simulink model "carga_on_off"  (R2024b)
settings: Solver=VariableStepAuto  StartTime=0.0  StopTime=10.0  RelTol=1e-3
undefined symbols (not defined in the file): bc_x, bc_y, H_c, Kc_y, M_s, M_x
settings Model: Creator=ribei  LastModifiedBy=ribei

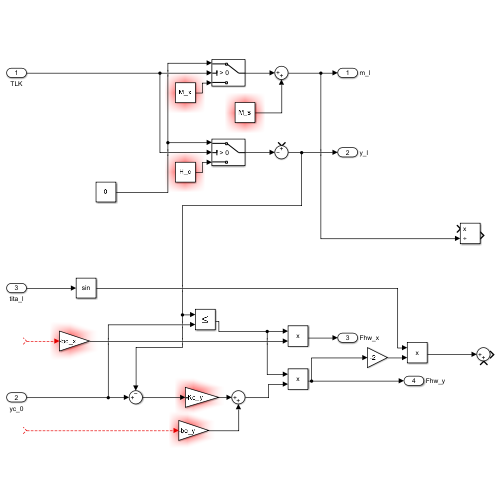
[thumbnail: Simulink's stored preview of the top-level diagram]
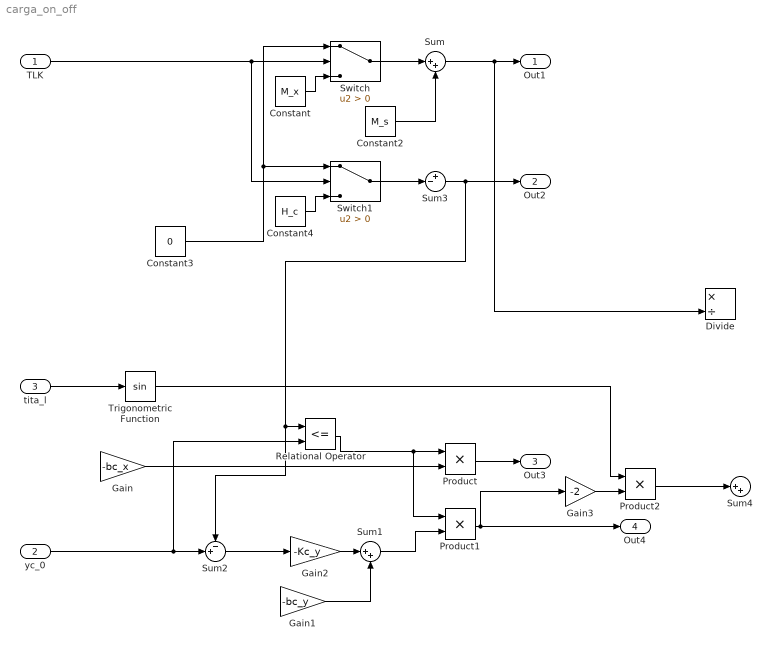
== system carga_on_off ==
  TLK : Inport
  yc_0 : Inport  Port=2
  tita_l : Inport  Port=3
  Constant : Constant  Value=M_x
  Constant2 : Constant  Value=M_s
  Constant3 : Constant  Value=0
  Constant4 : Constant  Value=H_c
  Divide : Product  Inputs=*/
  Gain : Gain  Gain=-bc_x
  Gain1 : Gain  Gain=-bc_y
  Gain2 : Gain  Gain=-Kc_y
  Gain3 : Gain  Gain=-2
  Product : Product
  Product1 : Product
  Product2 : Product
  Relational Operator : RelationalOperator  Operator=<=  OutDataTypeStr=boolean  RndMeth=Simplest  InputSameDT=off
  Sum : Sum  Inputs=|++
  Sum1 : Sum  Inputs=|++
  Sum2 : Sum  Inputs=-+|
  Sum3 : Sum  Inputs=+-|
  Sum4 : Sum  Inputs=|++
  Switch : Switch  Criteria=u2 > Threshold  SaturateOnIntegerOverflow=off  InputSameDT=off
  Switch1 : Switch  Criteria=u2 > Threshold  SaturateOnIntegerOverflow=off  InputSameDT=off
  Trigonometric Function : Trigonometry
  Out1 : Outport  SignalName=m_l
  Out2 : Outport  Port=2  SignalName=y_l
  Out3 : Outport  Port=3  SignalName=Fhw_x
  Out4 : Outport  Port=4  SignalName=Fhw_y
  wires:
  Switch/1 -> Sum/1
  Constant2/1 -> Sum/2
  Sum/1 -> Divide/2, Out1/1
  TLK/1 -> Switch/2, Switch1/2
  Constant/1 -> Switch/3
  Constant4/1 -> Switch1/3
  Switch1/1 -> Sum3/2
  Constant3/1 -> Switch1/1, Switch/1
  Sum2/1 -> Gain2/1
  Sum3/1 -> Sum2/1, Relational Operator/1, Out2/1
  ? -> Gain/1
  ? -> Gain1/1
  Gain2/1 -> Sum1/1
  Gain1/1 -> Sum1/2
  yc_0/1 -> Relational Operator/2, Sum2/2
  Relational Operator/1 -> Product/1, Product1/1
  Sum1/1 -> Product1/2
  Product/1 -> Out3/1
  Gain/1 -> Product/2
  tita_l/1 -> Trigonometric Function/1
  Product1/1 -> Gain3/1, Out4/1
  Gain3/1 -> Product2/2
  Trigonometric Function/1 -> Product2/1
  Product2/1 -> Sum4/1
